simulink model "Model"  (R2022b)
settings: Solver=VariableStepAuto  StartTime=0.0  StopTime=20.0  RelTol=1e-3
libraries: mcbcontrolslib x6, slpidlib x3, mcbpositiondecoderlib x2, spsDCVoltageSourceLib x1, spsPermanentMagnetSynchronousMachineLib x1, mcbhdlpositiondecoderlib x1, spsUniversalBridgeLib x1, sps_lib x1
settings Model: Creator=ADMIN  LastModifiedBy=ADMIN
settings SolverCC: ZeroCrossAlgorithm=Adaptive
settings DebuggingCC: IgnoredZcDiagnostic=none  ParameterPrecisionLossMsg=none

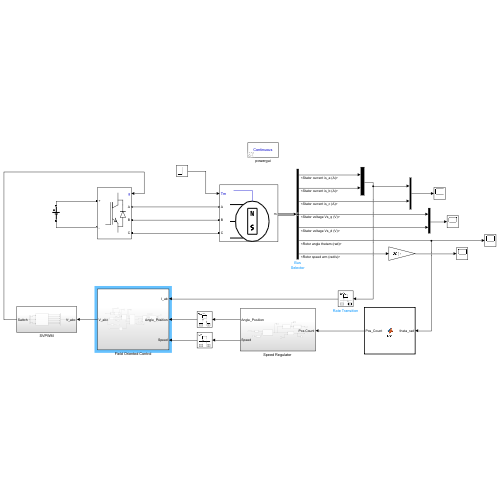
[thumbnail: Simulink's stored preview of the top-level diagram]
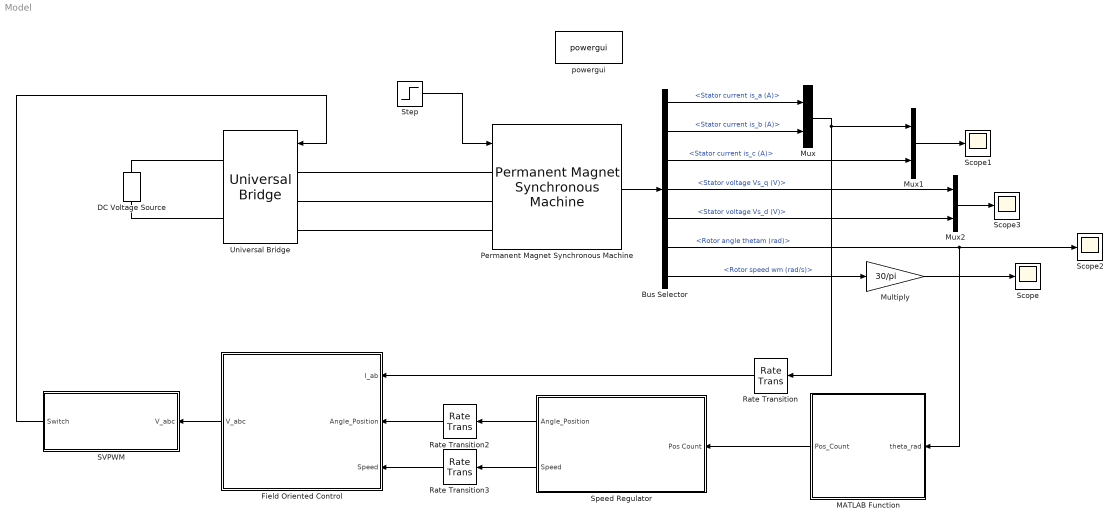
== system Model ==
  Bus Selector : BusSelector  OutputSignals=Stator current is_a (A),Stator current is_b (A),Stator current is_c (A),Stator voltage Vs_q (V),Stator voltage Vs_d (V),Rotor angle thetam (rad),Rotor speed wm (rad/s)
  DC Voltage Source : spsDCVoltageSourceLib/DC Voltage Source  Amplitude=48  Measurements=None
  Field Oriented Control : Subsystem
  MATLAB Function : MATLAB Function  TreatAsAtomicUnit=on
  Multiply : Gain  Gain=30/pi
  Mux : Mux  Inputs=2
  Mux1 : Mux  Inputs=2
  Mux2 : Mux  Inputs=2
  Permanent Magnet Synchronous Machine : spsPermanentMagnetSynchronousMachineLib/Permanent Magnet Synchronous Machine  NbPhases=3  FluxDistribution=Sinusoidal  RotorType=Round  MechanicalLoad=Torque Tm  PresetModel=No  ShowDetailedParameters=on  MeasurementBus=off  Resistance=0.105138  Inductance=8.5e-3  dqInductances=[8.5e-3,8.5e-3]  La=0.02  MachineConstant=Flux linkage established by magnets (V.s)  Flux=0.1194  VoltageCst=151.5974  TorqueCst=1.2537  Flat=120  Mechanical=[0.42 0.0004924 7 0.4]  PolePairs=4  InitialConditions=[0,0, 0,0]  InitialConditions5ph=[0 0 0 0 0 0]  RefAngle=90 degrees behind phase A axis (modified Park)  IterativeDiscreteModel=Trapezoidal non iterative  TsBlock=-1  TsPowergui=0
  Rate Transition : RateTransition
  Rate Transition2 : RateTransition
  Rate Transition3 : RateTransition
  SVPWM : Subsystem
  Scope{,1..3} (4 alike) : Scope
  "Speed Regulator " : Subsystem
  Step : Step  After=5  SampleTime=0
  Universal Bridge : spsUniversalBridgeLib/Universal Bridge  Arms=3  SnubberResistance=1e5  SnubberCapacitance=inf  Device=IGBT / Diodes  Ron=1e-3  Lon=0  ForwardVoltages="[  0  0  ]"  ForwardVoltage=0  GTOparameters=[ 10e-6 , 20e-6 ]  IGBTparameters=[ 1e-6 , 2e-6 ]  Measurements=None  Measurements_2=None  converterType=Rectifier
  powergui : sps_lib/powergui  Priority=1  SimulationMode=Continuous  SampleTime=5e-5  frequency=60  Iterations=50  frequencyindice=0  Pbase=100e6  ErrMax=1e-4  UnitsV=kV  UnitsW=MW  buscounter=0  FunctionMessages=off  echomessages=off  EnableUseOfTLC=off  CurrentSourceSwitches=off  DisableSnubberDevices=off  DisableRonSwitches=off  DisableVfSwitches=off  DisplayEquations=off  AutomaticDiscreteSolvers=off  SolverType=Tustin/Backward Euler (TBE)  Interpol=off  ExternalGateDelay=off  methode=off  Ts=100  x0status=blocks  SPID=on  SwTol=0  HookPort=off  NonlinearTolerance=1e-4  nMaxIteration=100  ContinueOnMaxIteration=off  RestoreLinks=warning  ResistiveCurrentMeasurement=off  Frange=[0:2:500]  Ylog=off  Xlog=on  ShowGrid=off  save=off  variable=ZData  structure=0  ZoomFFT=off  StartTime=0.0  cycles=1  DisplayStyle=1  fundamental=60  FreqAxis=off  MaxFrequency=1000  frequencyindicesteady=1  RmsSteady=1  display=off
  wires:
  "Speed Regulator "/2(Speed) -> Rate Transition3/1
  "Speed Regulator "/1(Angle_Position) -> Rate Transition2/1
  Permanent Magnet Synchronous Machine/1 -> Bus Selector/1
  Bus Selector/1 -> Mux/1  "<Stator current is_a (A)>"
  Bus Selector/2 -> Mux/2  "<Stator current is_b (A)>"
  Mux/1 -> Rate Transition/1, Mux1/1
  Bus Selector/7 -> Multiply/1  "<Rotor speed wm (rad/s)>"
  Multiply/1 -> Scope/1
  Rate Transition/1 -> Field Oriented Control/1(I_ab)
  Rate Transition2/1 -> Field Oriented Control/2(Angle_Position)
  Rate Transition3/1 -> Field Oriented Control/3(Speed)
  Bus Selector/3 -> Mux1/2  "<Stator current is_c (A)>"
  Mux1/1 -> Scope1/1
  Field Oriented Control/1(V_abc) -> SVPWM/1(V_abc)
  SVPWM/1(Switch) -> Universal Bridge/1
  Step/1 -> Permanent Magnet Synchronous Machine/1
  Bus Selector/6 -> Scope2/1, MATLAB Function/1(theta_rad)  "<Rotor angle thetam (rad)>"
  MATLAB Function/1(Pos_Count) -> "Speed Regulator "/1(Pos Count)
  Bus Selector/4 -> Mux2/1  "<Stator voltage Vs_q (V)>"
  Bus Selector/5 -> Mux2/2  "<Stator voltage Vs_d (V)>"
  Mux2/1 -> Scope3/1
  connections:
  Permanent Magnet Synchronous Machine/LConn1 -- Universal Bridge/LConn1
  Permanent Magnet Synchronous Machine/LConn2 -- Universal Bridge/LConn2
  Permanent Magnet Synchronous Machine/LConn3 -- Universal Bridge/LConn3
  DC Voltage Source/RConn1 -- Universal Bridge/RConn1
  DC Voltage Source/LConn1 -- Universal Bridge/RConn2

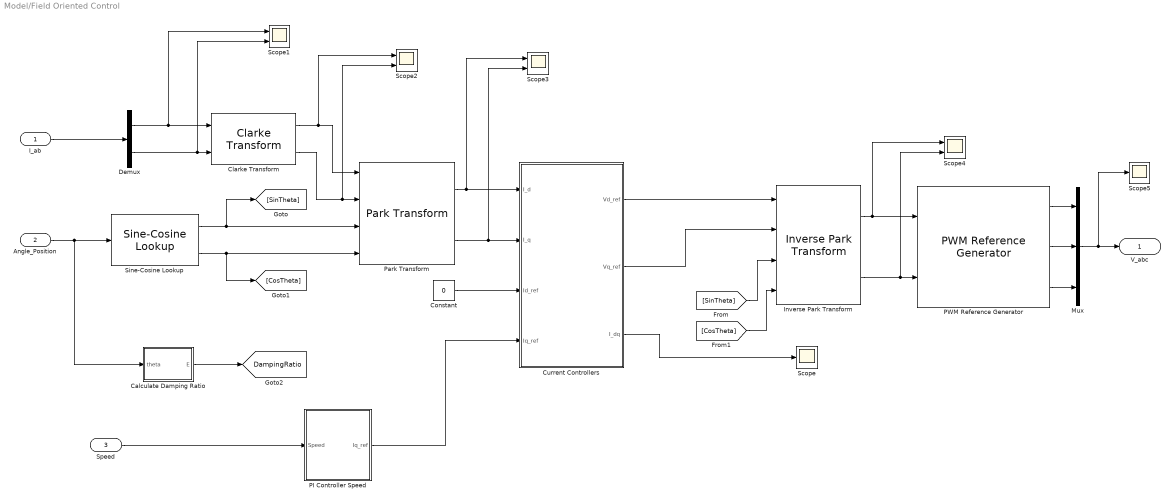
== system Model/Field Oriented Control ==
  I_ab : Inport
  Angle_Position : Inport  Port=2
  Speed : Inport  Port=3
  Calculate Damping Ratio : MATLAB Function  TreatAsAtomicUnit=on
  Clarke Transform : mcbcontrolslib/Clarke Transform  VariantControl=Variant2
      settings: LibrarySourceBlock=mcbhdllib/Controls/Math Transforms/Clarke Transform
  Constant : Constant  Value=0
  Current Controllers : Subsystem
  Demux : Demux  Outputs=2
  Inverse Park Transform : mcbcontrolslib/Inverse Park Transform  AxisAlignment=D-axis
      settings: LibrarySourceBlock=mcbhdllib/Controls/Math Transforms/Inverse Park Transform
  Mux : Mux  Inputs=3
  PI Controller Speed : Subsystem
  PWM Reference Generator : mcbcontrolslib/PWM Reference Generator  inSignal=Valphabeta  modType=SVM: space vector modulation
      settings: LibrarySourceBlock=mcbhdllib/Controls/Math Transforms/PWM Reference Generator
  Park Transform : mcbcontrolslib/Park Transform  AxisAlignment=D-axis
      settings: LibrarySourceBlock=mcbhdllib/Controls/Math Transforms/Park Transform
  Scope : Scope
  Scope{1..4} (4 alike) : Scope  NumInputPorts=2
  Scope5 : Scope
  Sine-Cosine Lookup : mcbcontrolslib/Sine-Cosine Lookup  AngleInput=Radians  N_points=1024
      settings: LibrarySourceBlock=mcblib/Controls/Math Transforms/Sine-Cosine Lookup
  V_abc : Outport
  tag scope: DampingRatio=global
  wires:
  Clarke Transform/1 -> Scope2/1, Park Transform/1
  Clarke Transform/2 -> Scope2/2, Park Transform/2
  Inverse Park Transform/1 -> Scope4/1, PWM Reference Generator/1
  Inverse Park Transform/2 -> Scope4/2, PWM Reference Generator/2
  Demux/1 -> Scope1/1, Clarke Transform/1
  Demux/2 -> Scope1/2, Clarke Transform/2
  Angle_Position/1 -> Calculate Damping Ratio/1(theta), Sine-Cosine Lookup/1
  Sine-Cosine Lookup/1 -> Park Transform/3, [SinTheta]
  Sine-Cosine Lookup/2 -> [CosTheta], Park Transform/4
  [SinTheta] -> Inverse Park Transform/3
  [CosTheta] -> Inverse Park Transform/4
  Park Transform/1 -> Scope3/1, Current Controllers/1(I_d)
  Park Transform/2 -> Scope3/2, Current Controllers/2(I_q)
  Current Controllers/1(Vd_ref) -> Inverse Park Transform/1
  Current Controllers/2(Vq_ref) -> Inverse Park Transform/2
  Current Controllers/3(I_dq) -> Scope/1
  Constant/1 -> Current Controllers/3(Id_ref)
  Speed/1 -> PI Controller Speed/1(Speed)
  I_ab/1 -> Demux/1
  PI Controller Speed/1(Iq_ref) -> Current Controllers/4(Iq_ref)
  Calculate Damping Ratio/1(E) -> [DampingRatio]
  PWM Reference Generator/2 -> Mux/2
  PWM Reference Generator/1 -> Mux/1
  PWM Reference Generator/3 -> Mux/3
  Mux/1 -> Scope5/1, V_abc/1

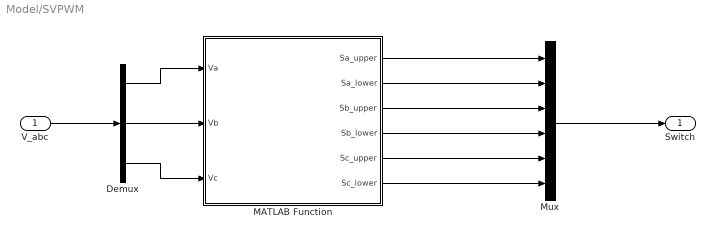
== system Model/SVPWM ==
  V_abc : Inport
  Demux : Demux  Outputs=3
  MATLAB Function : MATLAB Function  TreatAsAtomicUnit=on
  Mux : Mux  Inputs=6
  Switch : Outport
  wires:
  V_abc/1 -> Demux/1
  Demux/1 -> MATLAB Function/1(Va)
  Demux/2 -> MATLAB Function/2(Vb)
  Demux/3 -> MATLAB Function/3(Vc)
  MATLAB Function/3(Sb_upper) -> Mux/3
  MATLAB Function/2(Sa_lower) -> Mux/2
  MATLAB Function/1(Sa_upper) -> Mux/1
  MATLAB Function/4(Sb_lower) -> Mux/4
  MATLAB Function/5(Sc_upper) -> Mux/5
  MATLAB Function/6(Sc_lower) -> Mux/6
  Mux/1 -> Switch/1

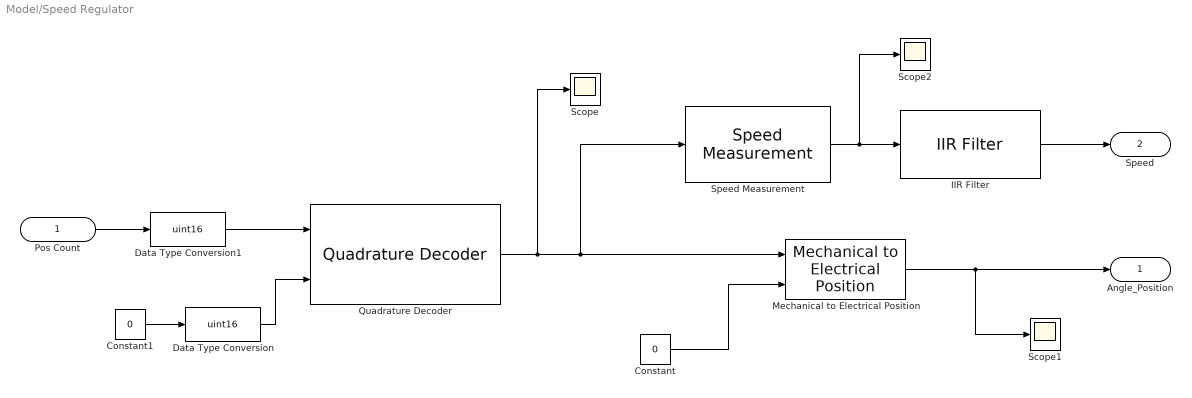
== system Model/Speed Regulator  ==
  Pos Count : Inport
  Constant : Constant  Value=0  SampleTime=-1
  Constant1 : Constant  Value=0  SampleTime=-1
  Data Type Conversion : DataTypeConversion  OutDataTypeStr=uint16  SaturateOnIntegerOverflow=off  RndMeth=Floor
  Data Type Conversion1 : DataTypeConversion  OutDataTypeStr=uint16  SaturateOnIntegerOverflow=off  RndMeth=Floor
  IIR Filter : mcbcontrolslib/IIR Filter  VariantControl=Low Pass Filter  VariantSelect=Low-pass  Filter_constant=0.01  advancedSettings=off  Ts=50e-6  cutOff_freq=32.1525
      settings: LibrarySourceBlock=mcblib/Signal Management/IIR Filter
  Mechanical to Electrical Position : mcbhdlpositiondecoderlib/Mechanical to Electrical Position  NrPP=7  selectedRange=Radians  MechOfstInputType=Input port  mechOffsetIn=0  maxAngleIn=2*pi  InputDataType=double  VariantSelect=floating-point
      settings: LibrarySourceBlock=mcbhdllib/Sensor Decoders/Mechanical to Electrical Position
  Quadrature Decoder : mcbpositiondecoderlib/Quadrature Decoder  EncoderSlitsPerRevolution=1000  EncoderCountsPerSlit=4  CounterSize=16 bits  ExternalIndexCount=on  PositionUnit=Radians  PositionDataType=single
      settings: LibrarySourceBlock=mcbhdllib/Sensor Decoders/Quadrature Decoder
  Scope : Scope
  Scope1 : Scope
  Scope2 : Scope
  Speed Measurement : mcbpositiondecoderlib/Speed Measurement  PositionUnit=Radians  PositionScalingDatatype=uint16  SpeedCalculationMode=Maximum application speed  SampleTimeAsync=100e-6  MaximumApplicationSpeed=4000  SpeedResolution=5e-6  DelayLength=74  MaximumMeasurableSpeed=4000  MeasurableSpeedResolution=0.12207  SpeedUnit=Radians/Sec  PerUnitSpeed=1000  SpeedDataType=single
      settings: LibrarySourceBlock=mcbhdllib/Sensor Decoders/Speed Measurement
  Angle_Position : Outport
  Speed : Outport  Port=2
  wires:
  Quadrature Decoder/1 -> Scope/1, Mechanical to Electrical Position/1, Speed Measurement/1
  Speed Measurement/1 -> Scope2/1, IIR Filter/1
  IIR Filter/1 -> Speed/1
  Mechanical to Electrical Position/1 -> Scope1/1, Angle_Position/1
  Constant/1 -> Mechanical to Electrical Position/2
  Constant1/1 -> Data Type Conversion/1
  Data Type Conversion/1 -> Quadrature Decoder/2
  Pos Count/1 -> Data Type Conversion1/1
  Data Type Conversion1/1 -> Quadrature Decoder/1

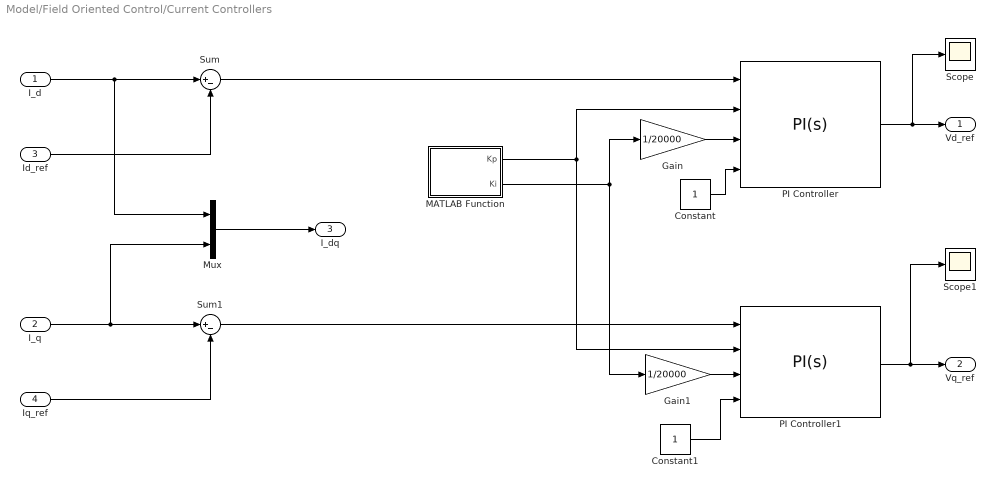
== system Model/Field Oriented Control/Current Controllers ==
  I_d : Inport
  I_q : Inport  Port=2
  Id_ref : Inport  Port=3
  Iq_ref : Inport  Port=4
  Constant : Constant
  Constant1 : Constant
  Gain : Gain  Gain=1/20000
  Gain1 : Gain  Gain=1/20000
  MATLAB Function : MATLAB Function  TreatAsAtomicUnit=on
  Mux : Mux  Inputs=2
  PI Controller : slpidlib/PID Controller  Controller=PI  Form=Parallel  TimeDomain=Continuous-time  UseExternalTs=off  SampleTime=-1  IntegratorMethod=Forward Euler  FilterMethod=Forward Euler  ControllerParametersSource=external  P=1  I=1  UseKiTs=on  D=0  N=100  UseFilter=on  TunerSelectOption=Transfer Function Based (PID Tuner App)  InitialConditionSource=internal  InitialConditionForIntegrator=0  InitialConditionForFilter=0  DifferentiatorICPrevScaledInput=0  ExternalReset=level  TrackingMode=off  Kt=1  LimitOutput=on  SatLimitsSource=internal  UpperSaturationLimit=1  LowerSaturationLimit=-1  LinearizeAsGain=on  AntiWindupMode=clamping  Kb=1  LimitIntegrator=off  UpperIntegratorSaturationLimit=inf  LowerIntegratorSaturationLimit=-inf  RndMeth=Simplest  POutMin=[]  POutMax=[]  IOutMin=[]  IOutMax=[]  DOutMin=[]  DOutMax=[]  NOutMin=[]  NOutMax=[]  SumOutMin=[]  SumOutMax=[]  SaturationOutDataTypeStr=Inherit: Inherit via back propagation  SaturationOutMin=[]  SaturationOutMax=[]  PParamMin=[]  PParamMax=[]  IParamMin=[]  IParamMax=[]  DParamMin=[]  DParamMax=[]  NParamMin=[]  NParamMax=[]  KbParamMin=[]  KbParamMax=[]  KtParamMin=[]  KtParamMax=[]  KbOutMin=[]  KbOutMax=[]  KtOutMin=[]  KtOutMax=[]  IntegratorOutMin=[]  IntegratorOutMax=[]  FilterOutMin=[]  FilterOutMax=[]  SumI1OutMin=[]  SumI1OutMax=[]  SumI2OutMin=[]  SumI2OutMax=[]  SumI3OutMin=[]  SumI3OutMax=[]  SumI4OutMin=[]  SumI4OutMax=[]  SumDOutMin=[]  SumDOutMax=[]  DifferentiatorOutMin=[]  DifferentiatorOutMax=[]  FilterDiffOutCoefMin=[]  FilterDiffOutCoefMax=[]  ReciprocalOutMin=[]  ReciprocalOutMax=[]  SumDenOutMin=[]  SumDenOutMax=[]  SumNumOutMin=[]  SumNumOutMax=[]  DivideOutMin=[]  DivideOutMax=[]  UdiffTsProdOutMin=[]  UdiffTsProdOutMax=[]  NTsProdOutMin=[]  NTsProdOutMax=[]  UintegralTsProdOutMin=[]  UintegralTsProdOutMax=[]  UngainTsProdOutMin=[]  UngainTsProdOutMax=[]  ClampingZeroOutDataTypeStr=Inherit: Inherit via back propagation  ClampingZeroOutMin=[]  ClampingZeroOutMax=[]  FilterDenConstantOutDataTypeStr=Inherit: Inherit via back propagation  FilterDenConstantOutMin=[]  FilterDenConstantOutMax=[]  PCopyOutDataTypeStr=Inherit: Inherit via back propagation  PCopyOutMin=[]  PCopyOutMax=[]  NCopyOutDataTypeStr=Inherit: Inherit via back propagation  NCopyOutMin=[]  NCopyOutMax=[]  IntegratorContinuousStateAttributes=''  IntegratorStateMustResolveToSignalObject=off  IntegratorRTWStateStorageClass=Auto  FilterContinuousStateAttributes=''  FilterStateMustResolveToSignalObject=off  FilterRTWStateStorageClass=Auto  ParallelPVariant=ExternalParameters  IdealPVariant=Disabled  IVariant=ExternalParameters  DVariant=Disabled  IntegratorVariant=Continuous  SatVariant=Enabled  AWVariant=ContClampingParallel  PCopyVariant=Disabled  TRVariant=Disabled  FdbkBlocksVariant=Forward  IdealPFdbkVariant=Disabled  SatFdbkVariant=Disabled  DerivativeFilterVariant=Disabled  NVariant=Disabled  NCopyVariant=Disabled_SignalSpec  FilterICVariant=Disabled  IntegratorICVariant=InternalICs  ExternalResetVariant=ExternalReset  TRSumVariant=Passthrough  SumFdbkVariant=Disabled  SumVariant=Sum_PI  TsampFilterVariant=InternalTs  TsampNgainVariant=Passthrough  TsampIntegralVariant=Passthrough  ExternalSaturationOutDataTypeStr=Inherit: Same as second input
      settings: LibrarySourceBlock=mcbhdllib/Controls/Controllers/PI Controller
  PI Controller1 : slpidlib/PID Controller  Controller=PI  Form=Parallel  TimeDomain=Continuous-time  UseExternalTs=off  SampleTime=-1  IntegratorMethod=Forward Euler  FilterMethod=Forward Euler  ControllerParametersSource=external  P=1  I=1  UseKiTs=on  D=0  N=100  UseFilter=on  TunerSelectOption=Transfer Function Based (PID Tuner App)  InitialConditionSource=internal  InitialConditionForIntegrator=0  InitialConditionForFilter=0  DifferentiatorICPrevScaledInput=0  ExternalReset=level  TrackingMode=off  Kt=1  LimitOutput=on  SatLimitsSource=internal  UpperSaturationLimit=1  LowerSaturationLimit=-1  LinearizeAsGain=on  AntiWindupMode=clamping  Kb=1  LimitIntegrator=off  UpperIntegratorSaturationLimit=inf  LowerIntegratorSaturationLimit=-inf  RndMeth=Simplest  POutMin=[]  POutMax=[]  IOutMin=[]  IOutMax=[]  DOutMin=[]  DOutMax=[]  NOutMin=[]  NOutMax=[]  SumOutMin=[]  SumOutMax=[]  SaturationOutDataTypeStr=Inherit: Inherit via back propagation  SaturationOutMin=[]  SaturationOutMax=[]  PParamMin=[]  PParamMax=[]  IParamMin=[]  IParamMax=[]  DParamMin=[]  DParamMax=[]  NParamMin=[]  NParamMax=[]  KbParamMin=[]  KbParamMax=[]  KtParamMin=[]  KtParamMax=[]  KbOutMin=[]  KbOutMax=[]  KtOutMin=[]  KtOutMax=[]  IntegratorOutMin=[]  IntegratorOutMax=[]  FilterOutMin=[]  FilterOutMax=[]  SumI1OutMin=[]  SumI1OutMax=[]  SumI2OutMin=[]  SumI2OutMax=[]  SumI3OutMin=[]  SumI3OutMax=[]  SumI4OutMin=[]  SumI4OutMax=[]  SumDOutMin=[]  SumDOutMax=[]  DifferentiatorOutMin=[]  DifferentiatorOutMax=[]  FilterDiffOutCoefMin=[]  FilterDiffOutCoefMax=[]  ReciprocalOutMin=[]  ReciprocalOutMax=[]  SumDenOutMin=[]  SumDenOutMax=[]  SumNumOutMin=[]  SumNumOutMax=[]  DivideOutMin=[]  DivideOutMax=[]  UdiffTsProdOutMin=[]  UdiffTsProdOutMax=[]  NTsProdOutMin=[]  NTsProdOutMax=[]  UintegralTsProdOutMin=[]  UintegralTsProdOutMax=[]  UngainTsProdOutMin=[]  UngainTsProdOutMax=[]  ClampingZeroOutDataTypeStr=Inherit: Inherit via back propagation  ClampingZeroOutMin=[]  ClampingZeroOutMax=[]  FilterDenConstantOutDataTypeStr=Inherit: Inherit via back propagation  FilterDenConstantOutMin=[]  FilterDenConstantOutMax=[]  PCopyOutDataTypeStr=Inherit: Inherit via back propagation  PCopyOutMin=[]  PCopyOutMax=[]  NCopyOutDataTypeStr=Inherit: Inherit via back propagation  NCopyOutMin=[]  NCopyOutMax=[]  IntegratorContinuousStateAttributes=''  IntegratorStateMustResolveToSignalObject=off  IntegratorRTWStateStorageClass=Auto  FilterContinuousStateAttributes=''  FilterStateMustResolveToSignalObject=off  FilterRTWStateStorageClass=Auto  ParallelPVariant=ExternalParameters  IdealPVariant=Disabled  IVariant=ExternalParameters  DVariant=Disabled  IntegratorVariant=Continuous  SatVariant=Enabled  AWVariant=ContClampingParallel  PCopyVariant=Disabled  TRVariant=Disabled  FdbkBlocksVariant=Forward  IdealPFdbkVariant=Disabled  SatFdbkVariant=Disabled  DerivativeFilterVariant=Disabled  NVariant=Disabled  NCopyVariant=Disabled_SignalSpec  FilterICVariant=Disabled  IntegratorICVariant=InternalICs  ExternalResetVariant=ExternalReset  TRSumVariant=Passthrough  SumFdbkVariant=Disabled  SumVariant=Sum_PI  TsampFilterVariant=InternalTs  TsampNgainVariant=Passthrough  TsampIntegralVariant=Passthrough  ExternalSaturationOutDataTypeStr=Inherit: Same as second input
      settings: LibrarySourceBlock=mcbhdllib/Controls/Controllers/PI Controller
  Scope : Scope
  Scope1 : Scope
  Sum : Sum  Inputs=|+-
  Sum1 : Sum  Inputs=|+-
  Vd_ref : Outport
  Vq_ref : Outport  Port=2
  I_dq : Outport  Port=3
  wires:
  I_d/1 -> Mux/1, Sum/1
  Id_ref/1 -> Sum/2
  Iq_ref/1 -> Sum1/2
  I_q/1 -> Mux/2, Sum1/1
  Mux/1 -> I_dq/1
  Sum/1 -> PI Controller/1
  PI Controller/1 -> Scope/1, Vd_ref/1
  Sum1/1 -> PI Controller1/1
  PI Controller1/1 -> Scope1/1, Vq_ref/1
  Constant/1 -> PI Controller/4
  Constant1/1 -> PI Controller1/4
  MATLAB Function/1(Kp) -> PI Controller1/2, PI Controller/2
  Gain/1 -> PI Controller/3
  MATLAB Function/2(Ki) -> Gain1/1, Gain/1
  Gain1/1 -> PI Controller1/3

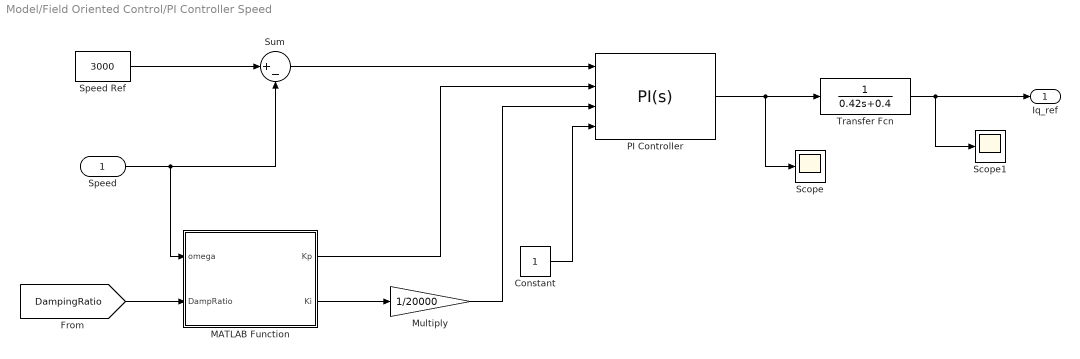
== system Model/Field Oriented Control/PI Controller Speed ==
  Speed : Inport
  Constant : Constant
  MATLAB Function : MATLAB Function  TreatAsAtomicUnit=on
  Multiply : Gain  Gain=1/20000
  PI Controller : slpidlib/PID Controller  Controller=PI  Form=Parallel  TimeDomain=Continuous-time  UseExternalTs=off  SampleTime=-1  IntegratorMethod=Forward Euler  FilterMethod=Forward Euler  ControllerParametersSource=external  P=1  I=1  UseKiTs=on  D=0  N=100  UseFilter=on  TunerSelectOption=Transfer Function Based (PID Tuner App)  InitialConditionSource=internal  InitialConditionForIntegrator=0  InitialConditionForFilter=0  DifferentiatorICPrevScaledInput=0  ExternalReset=level  TrackingMode=off  Kt=1  LimitOutput=on  SatLimitsSource=internal  UpperSaturationLimit=1  LowerSaturationLimit=-1  LinearizeAsGain=on  AntiWindupMode=clamping  Kb=1  LimitIntegrator=off  UpperIntegratorSaturationLimit=inf  LowerIntegratorSaturationLimit=-inf  RndMeth=Simplest  POutMin=[]  POutMax=[]  IOutMin=[]  IOutMax=[]  DOutMin=[]  DOutMax=[]  NOutMin=[]  NOutMax=[]  SumOutMin=[]  SumOutMax=[]  SaturationOutDataTypeStr=Inherit: Inherit via back propagation  SaturationOutMin=[]  SaturationOutMax=[]  PParamMin=[]  PParamMax=[]  IParamMin=[]  IParamMax=[]  DParamMin=[]  DParamMax=[]  NParamMin=[]  NParamMax=[]  KbParamMin=[]  KbParamMax=[]  KtParamMin=[]  KtParamMax=[]  KbOutMin=[]  KbOutMax=[]  KtOutMin=[]  KtOutMax=[]  IntegratorOutMin=[]  IntegratorOutMax=[]  FilterOutMin=[]  FilterOutMax=[]  SumI1OutMin=[]  SumI1OutMax=[]  SumI2OutMin=[]  SumI2OutMax=[]  SumI3OutMin=[]  SumI3OutMax=[]  SumI4OutMin=[]  SumI4OutMax=[]  SumDOutMin=[]  SumDOutMax=[]  DifferentiatorOutMin=[]  DifferentiatorOutMax=[]  FilterDiffOutCoefMin=[]  FilterDiffOutCoefMax=[]  ReciprocalOutMin=[]  ReciprocalOutMax=[]  SumDenOutMin=[]  SumDenOutMax=[]  SumNumOutMin=[]  SumNumOutMax=[]  DivideOutMin=[]  DivideOutMax=[]  UdiffTsProdOutMin=[]  UdiffTsProdOutMax=[]  NTsProdOutMin=[]  NTsProdOutMax=[]  UintegralTsProdOutMin=[]  UintegralTsProdOutMax=[]  UngainTsProdOutMin=[]  UngainTsProdOutMax=[]  ClampingZeroOutDataTypeStr=Inherit: Inherit via back propagation  ClampingZeroOutMin=[]  ClampingZeroOutMax=[]  FilterDenConstantOutDataTypeStr=Inherit: Inherit via back propagation  FilterDenConstantOutMin=[]  FilterDenConstantOutMax=[]  PCopyOutDataTypeStr=Inherit: Inherit via back propagation  PCopyOutMin=[]  PCopyOutMax=[]  NCopyOutDataTypeStr=Inherit: Inherit via back propagation  NCopyOutMin=[]  NCopyOutMax=[]  IntegratorContinuousStateAttributes=''  IntegratorStateMustResolveToSignalObject=off  IntegratorRTWStateStorageClass=Auto  FilterContinuousStateAttributes=''  FilterStateMustResolveToSignalObject=off  FilterRTWStateStorageClass=Auto  ParallelPVariant=ExternalParameters  IdealPVariant=Disabled  IVariant=ExternalParameters  DVariant=Disabled  IntegratorVariant=Continuous  SatVariant=Enabled  AWVariant=ContClampingParallel  PCopyVariant=Disabled  TRVariant=Disabled  FdbkBlocksVariant=Forward  IdealPFdbkVariant=Disabled  SatFdbkVariant=Disabled  DerivativeFilterVariant=Disabled  NVariant=Disabled  NCopyVariant=Disabled_SignalSpec  FilterICVariant=Disabled  IntegratorICVariant=InternalICs  ExternalResetVariant=ExternalReset  TRSumVariant=Passthrough  SumFdbkVariant=Disabled  SumVariant=Sum_PI  TsampFilterVariant=InternalTs  TsampNgainVariant=Passthrough  TsampIntegralVariant=Passthrough  ExternalSaturationOutDataTypeStr=Inherit: Same as second input
      settings: LibrarySourceBlock=mcbhdllib/Controls/Controllers/PI Controller
  Scope : Scope
  Scope1 : Scope
  Speed Ref : Constant  Value=3000  SampleTime=-1
  Sum : Sum  Inputs=|+-
  Transfer Fcn : TransferFcn  Denominator=[0.42 0.4]
  Iq_ref : Outport
  wires:
  Speed Ref/1 -> Sum/1
  Speed/1 -> MATLAB Function/1(omega), Sum/2
  Transfer Fcn/1 -> Scope1/1, Iq_ref/1
  Sum/1 -> PI Controller/1
  PI Controller/1 -> Scope/1, Transfer Fcn/1
  Constant/1 -> PI Controller/4
  [DampingRatio] -> MATLAB Function/2(DampRatio)
  MATLAB Function/1(Kp) -> PI Controller/2
  MATLAB Function/2(Ki) -> Multiply/1
  Multiply/1 -> PI Controller/3

== matlab function Model/Field Oriented Control/PI Controller Speed/MATLAB Function ==
  data: omega input; Kp output; Ki output; DampRatio input
function [Kp,Ki] = fcn(omega,DampRatio)

J = 0.42;

B = 0.4; 

Kp = 2 * DampRatio * omega * J * B;

Ki = J * omega;

== matlab function Model/Field Oriented Control/Calculate Damping Ratio ==
  data: theta input; E output
function E = fcn(theta)

E = sqrt(1 / ((tan(theta)^2 + 1)));

== matlab function Model/Field Oriented Control/Current Controllers/MATLAB Function ==
  data: Kp output; Ki output
function [Kp, Ki] = fcn()

%Khai báo constant

L = 0.02;

R = 0.1051;

f = 20000;

w0 = 2*pi*f;

zeta = 1;

Kp = 2*zeta*w0*(L-R);

Ki = Kp*(L*w0^2);

== matlab function Model/SVPWM/MATLAB Function ==
  data: Va input; Sa_upper output; Vb input; Vc input; Sa_lower output; Sb_upper output; Sb_lower output; Sc_upper output; Sc_lower output
function [Sa_upper, Sa_lower, Sb_upper, Sb_lower, Sc_upper, Sc_lower]  = fcn(Va, Vb, Vc)

%Deadtime = 0;
Ts = 1/20000;
Vdc = 48;


% Biến đổi Clarke: abc -> alpha-beta
Valpha = (2/3) * (Va - 0.5*Vb - 0.5*Vc);
Vbeta = (2/3) * (0.866*Vb - 0.866*Vc);

% Tính góc và biên độ vector điện áp tham chiếu
theta = atan2(Vbeta, Valpha);
if theta < 0
    theta = theta + 2*pi;
end

Vref = sqrt(Valpha^2 + Vbeta^2);

% Xác định Sector (1-6)
Sector = floor(theta / (pi/3)) + 1;
if Sector > 6
    Sector = 6;
end

% Tính góc trong sector (0 đến 60 độ)
theta_sector = theta - (Sector - 1) * (pi/3);

% Tính thời gian vector cơ bản
% Vdc/sqrt(3) là điện áp tối đa có thể điều chế
Vmax = Vdc / sqrt(3);

% Tính T1 và T2 (thời gian vector kề)
T1 = (Ts * Vref / Vmax) * sin(pi/3 - theta_sector);
T2 = (Ts * Vref / Vmax) * sin(theta_sector);
T0 = Ts - T1 - T2;

% Giới hạn quá điều chế
if (T1 + T2) > Ts
    k = Ts / (T1 + T2);
    T1 = T1 * k;
    T2 = T2 * k;
    T0 = 0;
end

% Phân bổ thời gian zero vector
Tz1 = T0 / 2;

% Tính thời gian đóng khóa cho từng pha theo sector
% Sử dụng chuỗi đối xứng 7 đoạn: 0-1-2-7-2-1-0
switch Sector
    case 1
        Tcm1 = Tz1 + T1 + T2;
        Tcm2 = Tz1 + T2;
        Tcm3 = Tz1;
    case 2
        Tcm1 = Tz1 + T1;
        Tcm2 = Tz1 + T1 + T2;
        Tcm3 = Tz1;
    case 3
        Tcm1 = Tz1;
        Tcm2 = Tz1 + T1 + T2;
        Tcm3 = Tz1 + T2;
    case 4
        Tcm1 = Tz1;
        Tcm2 = Tz1 + T1;
        Tcm3 = Tz1 + T1 + T2;
    case 5
        Tcm1 = Tz1 + T2;
        Tcm2 = Tz1;
        Tcm3 = Tz1 + T1 + T2;
    case 6
        Tcm1 = Tz1 + T1 + T2;
        Tcm2 = Tz1;
        Tcm3 = Tz1 + T1;
    otherwise
        Tcm1 = 0;
        Tcm2 = 0;
        Tcm3 = 0;
end

% Chuẩn hóa thời gian đóng (duty cycle 0-1)
Ta = Tcm1 / Ts;
Tb = Tcm2 / Ts;
Tc = Tcm3 / Ts;

% Giới hạn duty cycle trong khoảng [0, 1]
Ta = max(0, min(1, Ta));
Tb = max(0, min(1, Tb));
Tc = max(0, min(1, Tc));

% Tạo tín hiệu cho khóa trên (upper switches)
Sa_upper = Ta;
Sb_upper = Tb;
Sc_upper = Tc;

% Tạo tín hiệu cho khóa dưới (lower switches)
% Khóa dưới bù với khóa trên (complementary) + deadtime
Sa_lower = 1 - Ta;
Sb_lower = 1 - Tb;
Sc_lower = 1 - Tc;

% Áp dụng deadtime nếu có
% if Deadtime > 0
%     deadtime_ratio = Deadtime / Ts;
%     
%     % Giảm duty cycle cho khóa trên
%     Sa_upper = max(0, Sa_upper - deadtime_ratio);
%     Sb_upper = max(0, Sb_upper - deadtime_ratio);
%     Sc_upper = max(0, Sc_upper - deadtime_ratio);
%     
%     % Giảm duty cycle cho khóa dưới
%     Sa_lower = max(0, Sa_lower - deadtime_ratio);
%     Sb_lower = max(0, Sb_lower - deadtime_ratio);
%     Sc_lower = max(0, Sc_lower - deadtime_ratio);
% end 

end

== matlab function Model/MATLAB Function ==
  data: theta_rad input; Pos_Count output
function Pos_Count = fcn(theta_rad)

CountsPerRev = 4096;  % số xung encoder trên một vòng (CPR)

theta_mod = mod(theta_rad, 2*pi);

% Tính số count
count_float = (theta_mod / (2*pi)) * CountsPerRev;

% Làm tròn và ép kiểu về uint16
Pos_Count = uint16(round(count_float));

end
